simulink model "freqconv"  (Simulink 10.3)
settings: Solver=ode23tb  StartTime=0.0  StopTime=0.1  MaxStep=5e-6  RelTol=1e-3  EnableMultiTasking=on
libraries: spsIGBTLib x4, spsVoltageMeasurementLib x2, spsACVoltageSourceLib x1, spsLinearTransformerLib x1, spsCurrentMeasurementLib x1, spsSeriesRLCBranchLib x1, spspowerguiLib x1
settings Model: Creator=kAnnanvalar  LastModifiedBy=Rahul
settings DataIOCC: LimitDataPoints=on
settings DebuggingCC: SolverPrmCheckMsg=warning

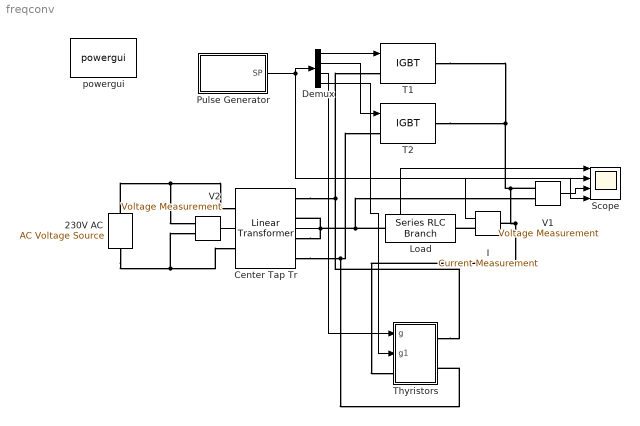
== system freqconv ==
  230V AC : spsACVoltageSourceLib/AC Voltage Source  Amplitude=230*sqrt(2)  Phase=0  Frequency=50  SampleTime=0  Measurements=None  BusType=swing  Pref=10e3  Qref=0  Qmin=-inf  Qmax=+inf
  Center Tap Tr : spsLinearTransformerLib/Linear Transformer  UNITS=pu  NominalPower=[ 10e3 100 ]  winding1="[ 230  0.002  0.08 ]"  winding2="[ 230  0.002  0.08 ]"  ThreeWindings=on  winding3=[ 230 0.002 0.08 ]  RmLm=[ 500 500 ]  Measurements=None  DataType=off
  Demux : Demux
  I : spsCurrentMeasurementLib/Current Measurement  PhasorSimulation=off  OutputType=Complex  PSBequivalent=0
  Load : spsSeriesRLCBranchLib/Series RLC Branch  LConnTagsString=__new0  RConnTagsString=__new0  BranchType=R  Resistance=10  Inductance=1e-3  SetiL0=off  InitialCurrent=0  Capacitance=1e-6  Setx0=off  InitialVoltage=0  Measurements=None
  Pulse Generator : Subsystem  mask{t=100, a=99}
      mask prompts: t "Enter the output fequency (in Hz)"; a "Enter the Output voltage (in %)"
  Scope : Scope  NumInputPorts=4
  T1 : spsIGBTLib/IGBT  Ron=0.001  Lon=0  Vf=1  Tf=1e-6  Tt=2e-6  IC=0  Rs=1e5  Cs=inf  Measurements=off
  T2 : spsIGBTLib/IGBT  Ron=0.001  Lon=0  Vf=1  Tf=1e-6  Tt=2e-6  IC=0  Rs=1e5  Cs=inf  Measurements=off
  Thyristors : Subsystem
  V1 : spsVoltageMeasurementLib/Voltage Measurement  PhasorSimulation=off  OutputType=Complex  PSBequivalent=0
  V2 : spsVoltageMeasurementLib/Voltage Measurement  PhasorSimulation=off  OutputType=Complex  PSBequivalent=0
  powergui : spspowerguiLib/powergui  Priority=1  SimulationMode=Discrete  SampleTime=5e-6  frequency=60  Iterations=50  frequencyindice=50  Pbase=100e6  ErrMax=1e-4  UnitsV=kV  UnitsW=MW  buscounter=0  FunctionMessages=off  echomessages=off  EnableUseOfTLC=off  CurrentSourceSwitches=off  DisableSnubberDevices=off  DisableRonSwitches=off  DisableVfSwitches=off  DisplayEquations=off  AutomaticDiscreteSolvers=off  SolverType=Tustin/Backward Euler (TBE)  Interpol=off  ExternalGateDelay=off  methode=off  Ts=0  x0status=blocks  SPID=off  SwTol=0  HookPort=off  NonlinearTolerance=1e-4  nMaxIteration=100  ContinueOnMaxIteration=off  RestoreLinks=warning  ResistiveCurrentMeasurement=off  Frange=[0:2:500]  Ylog=off  Xlog=on  ShowGrid=off  save=off  variable=ZData  structure=0  ZoomFFT=on  StartTime=0.0  cycles=1  DisplayStyle=1  fundamental=60  FreqAxis=off  MaxFrequency=1000  frequencyindicesteady=1  RmsSteady=1  display=off
  wires:
  V1/1 -> Scope/3
  V2/1 -> Scope/1
  Pulse Generator/1(SP) -> Scope/2, Demux/1
  Demux/1 -> T1/1
  Demux/2 -> T2/1
  I/1 -> Scope/4
  Demux/3 -> Thyristors/1(g)
  Demux/4 -> Thyristors/2(g1)
  connections:
  230V AC/RConn1 -- Center Tap Tr/LConn1 -- V2/LConn1
  230V AC/LConn1 -- Center Tap Tr/LConn2 -- V2/LConn2
  Center Tap Tr/RConn1 -- Thyristors/RConn1 -- T1/LConn1
  Center Tap Tr/RConn3 -- Load/LConn1 -- V1/LConn2 -- Center Tap Tr/RConn2
  Center Tap Tr/RConn4 -- Thyristors/RConn2 -- T2/LConn1
  I/RConn1 -- Load/RConn1
  V1/LConn1 -- T1/RConn1 -- T2/RConn1 -- Thyristors/LConn1 -- I/LConn1

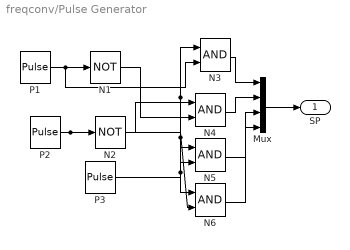
== system freqconv/Pulse Generator ==
  Mux : Mux
  N1 : Logic  Operator=NOT  AllPortsSameDT=off  OutDataTypeStr=boolean
  N2 : Logic  Operator=NOT  AllPortsSameDT=off  OutDataTypeStr=boolean
  N{3..6} (4 alike) : Logic  AllPortsSameDT=off  OutDataTypeStr=boolean
  P1 : DiscretePulseGenerator  PulseType=Time based  Period=(1/t)  PulseWidth=50
  P2 : DiscretePulseGenerator  PulseType=Time based  Period=(1/t)  PulseWidth=50  PhaseDelay=(1/t)/2
  P3 : DiscretePulseGenerator  PulseType=Time based  Period=1e-3  PulseWidth=a
  SP : Outport
  wires:
  P1/1 -> N1/1, N3/2
  P2/1 -> N2/1, N6/2
  N2/1 -> N4/2
  N1/1 -> N5/2
  Mux/1 -> SP/1
  N3/1 -> Mux/1
  N4/1 -> Mux/2
  N5/1 -> Mux/3
  N6/1 -> Mux/4
  P3/1 -> N6/1, N5/1, N3/1, N4/1

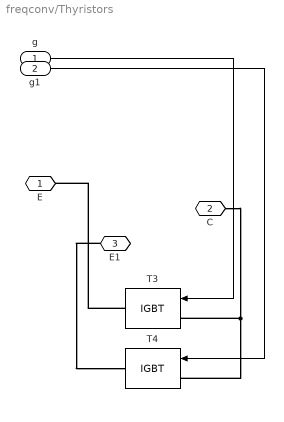
== system freqconv/Thyristors ==
  g : Inport
  g1 : Inport  Port=2
  T3 : spsIGBTLib/IGBT  Ron=0.001  Lon=0  Vf=1  Tf=1e-6  Tt=2e-6  IC=0  Rs=1e5  Cs=inf  Measurements=off
  T4 : spsIGBTLib/IGBT  Ron=0.001  Lon=0  Vf=1  Tf=1e-6  Tt=2e-6  IC=0  Rs=1e5  Cs=inf  Measurements=off
  E : PMIOPort  Side=Right
  C : PMIOPort  Port=2  Side=Left
  E1 : PMIOPort  Port=3  Side=Right
  wires:
  g1/1 -> T4/1
  g/1 -> T3/1
  connections:
  T4/LConn1 -- C/RConn1 -- T3/LConn1
  E1/RConn1 -- T4/RConn1
  T3/RConn1 -- E/RConn1
